simulink model "PMSMSimple"  (R2020a)
settings: Solver=VariableStepAuto  StartTime=0.0  StopTime=10.0  RelTol=1e-3
undefined symbols (not defined in the file or in its folder): n_pole_pairs, rotor_inertia, static_friction, torque_constant, viscous_damping
libraries: mcbcontrolslib x1, autolibpmsmexterior x1
settings Model: Creator=mahoyen  LastModifiedBy=mahoyen

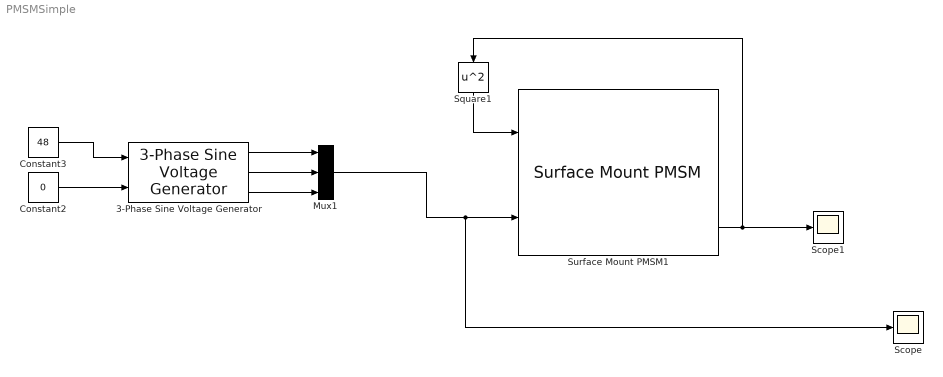
== system PMSMSimple ==
  3-Phase Sine Voltage Generator : mcbcontrolslib/3-Phase Sine Voltage Generator  AngleInput=Per-unit  N_points=1024
      settings: SourceProductBaseCode=MT
  Constant2 : Constant  Value=0
  Constant3 : Constant  Value=48
  Mux1 : Mux  Inputs=3
  Scope : Scope
  Scope1 : Scope
  Square1 : Math  Operator=square  SaturateOnIntegerOverflow=on
  Surface Mount PMSM1 : autolibpmsmexterior/Surface Mount PMSM  port_config=Torque  sim_type=Continuous  Ts=0.001  P=n_pole_pairs  Rs=stator_resistance  Ldq_=stator_inductance  KConstText=Torque constant (Kt):  lambda_pm=0.2205  Ke=159.9771  Kt=torque_constant  mechanical=[rotor_inertia, viscous_damping, static_friction]  idq0=[0 0]  theta_init=0  omega_init=0  KConst=torque_constant  lambda_pm_calc=0.001875  RefBlkName='autolibpmsmexterior/Surface Mount PMSM'  aMode=5  Ldq="[0.0017      0.0017]"
      settings: SourceProductBaseCode=PW,MT,VE,VP
  wires:
  Mux1/1 -> Scope/1, Surface Mount PMSM1/2
  Constant3/1 -> 3-Phase Sine Voltage Generator/1
  3-Phase Sine Voltage Generator/1 -> Mux1/1
  Square1/1 -> Surface Mount PMSM1/1
  Surface Mount PMSM1/3 -> Square1/1, Scope1/1
  3-Phase Sine Voltage Generator/2 -> Mux1/2
  Constant2/1 -> 3-Phase Sine Voltage Generator/2
  3-Phase Sine Voltage Generator/3 -> Mux1/3
